simulink model "tank_sandbox"  (R2016a)
settings: Solver=VariableStepAuto  StartTime=0.0  StopTime=10.0  RelTol=1e-3
libraries: tank_model x1
settings Model: Creator=Ibrahim  LastModifiedBy=Ibrahim

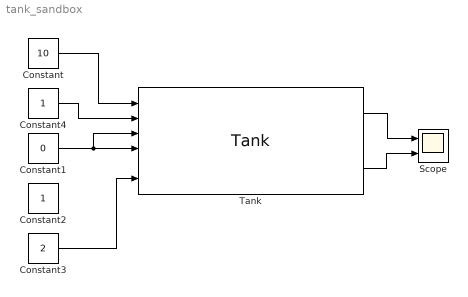
== system tank_sandbox ==
  Constant : Constant  Value=10
  Constant1 : Constant  Value=0
  Constant2 : Constant
  Constant3 : Constant  Value=2
  Constant4 : Constant
  Scope : Scope  NumInputPorts=2
  Tank : tank_model/Tank
  wires:
  Constant1/1 -> Tank/4, Tank/3
  Constant/1 -> Tank/1
  Tank/1 -> Scope/1
  Constant3/1 -> Tank/6
  Constant4/1 -> Tank/2
  Tank/2 -> Scope/2
